simulink model "BoucleVitesse"  (R2021a)
settings: Solver=VariableStepAuto  StartTime=0.0  StopTime=.1  RelTol=1e-3
values from neighbouring files (symbols this model uses):
  Jeq = 0.000022    (= 2.2e-05)    [param.m]
  Km = 0.0302    [param.m]
  L = 0.0000823    (= 8.23e-05)    [param.m]
  R = 0.299    [param.m]
settings Model: Creator=xpess  LastModifiedBy=xpess

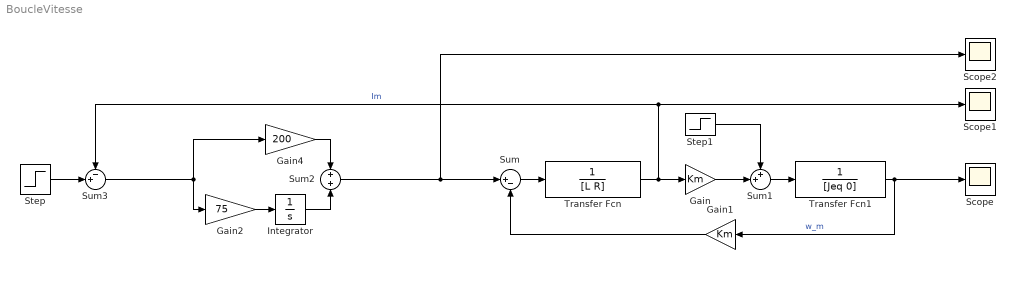
== system BoucleVitesse ==
  Gain : Gain  Gain=Km
  Gain1 : Gain  Gain=Km
  Gain2 : Gain  Gain=75
  Gain4 : Gain  Gain=200
  Integrator : Integrator
  Scope : Scope
  Scope1 : Scope
  Scope2 : Scope
  Step : Step  Time=0  SampleTime=0
  Step1 : Step  Time=0  After=0  SampleTime=0
  Sum : Sum  Inputs=|+-
  Sum1 : Sum  Inputs=++|
  Sum2 : Sum  Inputs=+|+
  Sum3 : Sum  Inputs=-+|
  Transfer Fcn : TransferFcn  Denominator=[L R]
  Transfer Fcn1 : TransferFcn  Denominator=[Jeq 0]
  wires:
  Transfer Fcn/1 -> Gain/1, Sum3/1, Scope1/1  "Im"
  Transfer Fcn1/1 -> Scope/1, Gain1/1  "w_m"
  Gain1/1 -> Sum/2
  Sum/1 -> Transfer Fcn/1
  Sum1/1 -> Transfer Fcn1/1
  Gain/1 -> Sum1/2
  Step1/1 -> Sum1/1
  Sum3/1 -> Gain4/1, Gain2/1
  Gain4/1 -> Sum2/1
  Integrator/1 -> Sum2/2
  Step/1 -> Sum3/2
  Sum2/1 -> Scope2/1, Sum/1
  Gain2/1 -> Integrator/1
